simulink library "INT_PTLo_LosCalc"  (R2016b)
settings: Solver=VariableStepAuto  StartTime=0.0  StopTime=10.0  RelTol=1e-3
settings Model: Creator=Administrator  LastModifiedBy=Administrator

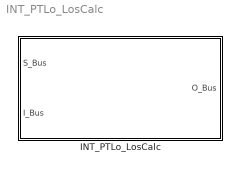
== system INT_PTLo_LosCalc ==
  INT_PTLo_LosCalc : Subsystem

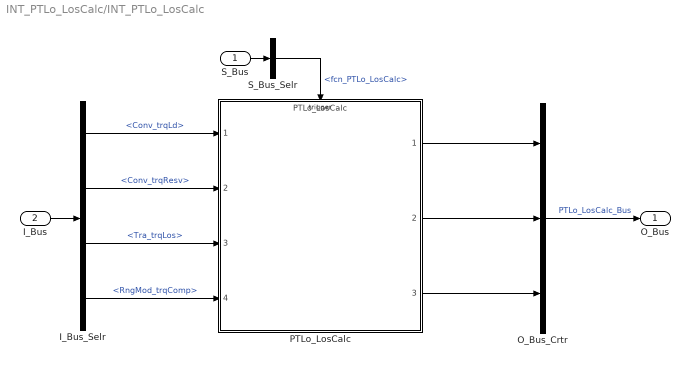
== system INT_PTLo_LosCalc/INT_PTLo_LosCalc ==
  S_Bus : Inport
  I_Bus : Inport  Port=2
  I_Bus_Selr : BusSelector  OutputSignals=Conv_trqLd,Conv_trqResv,Tra_trqLos,RngMod_trqComp
  O_Bus_Crtr : BusCreator  Inputs=3
  PTLo_LosCalc : ModelReference  ModelNameDialog=PTLo_LosCalc  SimulationMode=Normal  ModelReferenceVersion=1.2  TriggerPortName=function  TriggerPortTriggerType=function-call  TriggerPortStatesWhenEnabling=held
  S_Bus_Selr : BusSelector  OutputSignals=fcn_PTLo_LosCalc
  O_Bus : Outport
  wires:
  S_Bus_Selr/1 -> PTLo_LosCalc/Trigger  "<fcn_PTLo_LosCalc>"
  S_Bus/1 -> S_Bus_Selr/1
  I_Bus/1 -> I_Bus_Selr/1
  I_Bus_Selr/1 -> PTLo_LosCalc/1  "<Conv_trqLd>"
  I_Bus_Selr/2 -> PTLo_LosCalc/2  "<Conv_trqResv>"
  I_Bus_Selr/3 -> PTLo_LosCalc/3  "<Tra_trqLos>"
  I_Bus_Selr/4 -> PTLo_LosCalc/4  "<RngMod_trqComp>"
  O_Bus_Crtr/1 -> O_Bus/1  "PTLo_LosCalc_Bus"
  PTLo_LosCalc/1 -> O_Bus_Crtr/1
  PTLo_LosCalc/2 -> O_Bus_Crtr/2
  PTLo_LosCalc/3 -> O_Bus_Crtr/3
